simulink model "MHILSimRef"  (R2021b)
settings: Solver=VariableStepAuto  StartTime=0.0  StopTime=1e-3  RelTol=1e-3
values from neighbouring files (symbols this model uses):
  m = tddbl_model    [HILSimModel.m]
undefined symbols (not defined in the file or in its folder): s
libraries: simulink x3
settings Model: Creator=berndorfer  LastModifiedBy=berndorfer

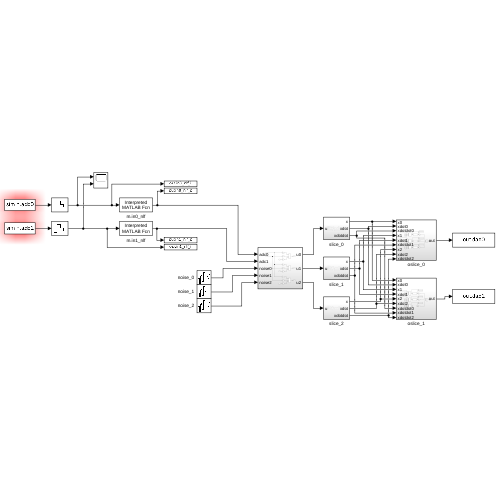
[thumbnail: Simulink's stored preview of the top-level diagram]
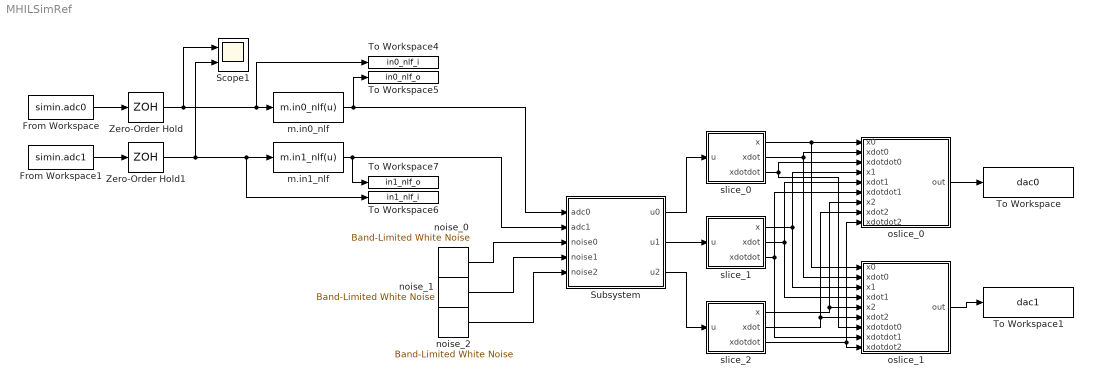
== system MHILSimRef ==
  From Workspace : FromWorkspace  VariableName=simin.adc0
  From Workspace1 : FromWorkspace  VariableName=simin.adc1
  Scope1 : Scope  NumInputPorts=2
  Subsystem : Subsystem
  To Workspace : ToWorkspace  VariableName=dac0  SaveFormat=Timeseries  SampleTime=-1
  To Workspace1 : ToWorkspace  VariableName=dac1  SaveFormat=Timeseries  SampleTime=-1
  To Workspace4 : ToWorkspace  VariableName=in0_nlf_i  SaveFormat=Timeseries  SampleTime=-1
  To Workspace5 : ToWorkspace  VariableName=in0_nlf_o  SaveFormat=Timeseries  SampleTime=-1
  To Workspace6 : ToWorkspace  VariableName=in1_nlf_i  SaveFormat=Timeseries  SampleTime=-1
  To Workspace7 : ToWorkspace  VariableName=in1_nlf_o  SaveFormat=Timeseries  SampleTime=-1
  Zero-Order Hold : ZeroOrderHold  SampleTime=m.t_s
  Zero-Order Hold1 : ZeroOrderHold  SampleTime=m.t_s
  m.in0_nlf : MATLABFcn  MATLABFcn=m.in0_nlf(u)  OutputDimensions=1
  m.in1_nlf : MATLABFcn  MATLABFcn=m.in1_nlf(u)  OutputDimensions=1
  noise_0 : simulink/Sources/Band-Limited White Noise  Cov=[m.n0_power*m.t_s]  Ts=m.t_s  seed=[23341]
  noise_1 : simulink/Sources/Band-Limited White Noise  Cov=[m.n1_power*m.t_s]  Ts=m.t_s  seed=[23341]
  noise_2 : simulink/Sources/Band-Limited White Noise  Cov=[m.n2_power*m.t_s]  Ts=m.t_s  seed=[23341]
  oslice_0 : Subsystem
  oslice_1 : Subsystem
  slice_0 : Subsystem
  slice_1 : Subsystem
  slice_2 : Subsystem
  wires:
  Subsystem/2(u1) -> slice_1/1(u)
  Subsystem/3(u2) -> slice_2/1(u)
  Subsystem/1(u0) -> slice_0/1(u)
  Zero-Order Hold/1 -> Scope1/1, To Workspace4/1, m.in0_nlf/1
  m.in1_nlf/1 -> Subsystem/2(adc1), To Workspace7/1
  noise_1/1 -> Subsystem/4(noise1)
  m.in0_nlf/1 -> Subsystem/1(adc0), To Workspace5/1
  noise_2/1 -> Subsystem/5(noise2)
  noise_0/1 -> Subsystem/3(noise0)
  Zero-Order Hold1/1 -> Scope1/2, To Workspace6/1, m.in1_nlf/1
  From Workspace/1 -> Zero-Order Hold/1
  From Workspace1/1 -> Zero-Order Hold1/1
  slice_1/1(x) -> oslice_1/3(x1), oslice_0/4(x1)
  slice_0/1(x) -> oslice_1/1(x0), oslice_0/1(x0)
  slice_2/2(xdot) -> oslice_0/8(xdot2), oslice_1/6(xdot2)
  slice_0/2(xdot) -> oslice_1/2(xdot0), oslice_0/2(xdot0)
  slice_2/1(x) -> oslice_1/5(x2), oslice_0/7(x2)
  slice_1/2(xdot) -> oslice_1/4(xdot1), oslice_0/5(xdot1)
  oslice_0/1(out) -> To Workspace/1
  oslice_1/1(out) -> To Workspace1/1
  slice_0/3(xdotdot) -> oslice_1/7(xdotdot0), oslice_0/3(xdotdot0)
  slice_1/3(xdotdot) -> oslice_1/8(xdotdot1), oslice_0/6(xdotdot1)
  slice_2/3(xdotdot) -> oslice_1/9(xdotdot2), oslice_0/9(xdotdot2)

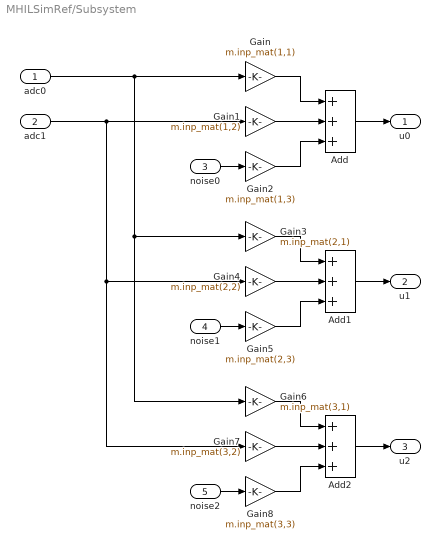
== system MHILSimRef/Subsystem ==
  adc0 : Inport
  adc1 : Inport  Port=2
  noise0 : Inport  Port=3
  noise1 : Inport  Port=4
  noise2 : Inport  Port=5
  Add : Sum  Inputs=+++
  Add1 : Sum  Inputs=+++
  Add2 : Sum  Inputs=+++
  Gain : Gain  Gain=m.inp_mat(1,1)
  Gain1 : Gain  Gain=m.inp_mat(1,2)
  Gain2 : Gain  Gain=m.inp_mat(1,3)
  Gain3 : Gain  Gain=m.inp_mat(2,1)
  Gain4 : Gain  Gain=m.inp_mat(2,2)
  Gain5 : Gain  Gain=m.inp_mat(2,3)
  Gain6 : Gain  Gain=m.inp_mat(3,1)
  Gain7 : Gain  Gain=m.inp_mat(3,2)
  Gain8 : Gain  Gain=m.inp_mat(3,3)
  u0 : Outport
  u1 : Outport  Port=2
  u2 : Outport  Port=3
  wires:
  adc0/1 -> Gain6/1, Gain3/1, Gain/1
  adc1/1 -> Gain7/1, Gain4/1, Gain1/1
  noise0/1 -> Gain2/1
  Gain1/1 -> Add/2
  Gain/1 -> Add/1
  Gain2/1 -> Add/3
  Add/1 -> u0/1
  noise1/1 -> Gain5/1
  Gain4/1 -> Add1/2
  Gain3/1 -> Add1/1
  Gain5/1 -> Add1/3
  Add1/1 -> u1/1
  noise2/1 -> Gain8/1
  Gain7/1 -> Add2/2
  Gain6/1 -> Add2/1
  Gain8/1 -> Add2/3
  Add2/1 -> u2/1

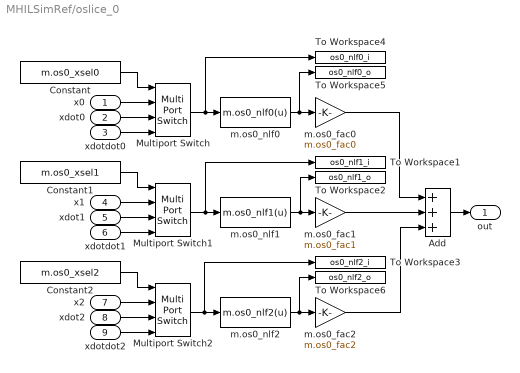
== system MHILSimRef/oslice_0 ==
  x0 : Inport
  xdot0 : Inport  Port=2
  xdotdot0 : Inport  Port=3
  x1 : Inport  Port=4
  xdot1 : Inport  Port=5
  xdotdot1 : Inport  Port=6
  x2 : Inport  Port=7
  xdot2 : Inport  Port=8
  xdotdot2 : Inport  Port=9
  Add : Sum  Inputs=+++
  Constant : Constant  Value=m.os0_xsel0
  Constant1 : Constant  Value=m.os0_xsel1
  Constant2 : Constant  Value=m.os0_xsel2
  Multiport Switch : MultiPortSwitch  DataPortOrder=Zero-based contiguous  zeroidx=on
  Multiport Switch1 : MultiPortSwitch  DataPortOrder=Zero-based contiguous  zeroidx=on
  Multiport Switch2 : MultiPortSwitch  DataPortOrder=Zero-based contiguous  zeroidx=on
  To Workspace1 : ToWorkspace  VariableName=os0_nlf1_i  SaveFormat=Timeseries  SampleTime=-1
  To Workspace2 : ToWorkspace  VariableName=os0_nlf1_o  SaveFormat=Timeseries  SampleTime=-1
  To Workspace3 : ToWorkspace  VariableName=os0_nlf2_i  SaveFormat=Timeseries  SampleTime=-1
  To Workspace4 : ToWorkspace  VariableName=os0_nlf0_i  SaveFormat=Timeseries  SampleTime=-1
  To Workspace5 : ToWorkspace  VariableName=os0_nlf0_o  SaveFormat=Timeseries  SampleTime=-1
  To Workspace6 : ToWorkspace  VariableName=os0_nlf2_o  SaveFormat=Timeseries  SampleTime=-1
  m.os0_fac0 : Gain  Gain=m.os0_fac0
  m.os0_fac1 : Gain  Gain=m.os0_fac1
  m.os0_fac2 : Gain  Gain=m.os0_fac2
  m.os0_nlf0 : MATLABFcn  MATLABFcn=m.os0_nlf0(u)  OutputDimensions=1
  m.os0_nlf1 : MATLABFcn  MATLABFcn=m.os0_nlf1(u)  OutputDimensions=1
  m.os0_nlf2 : MATLABFcn  MATLABFcn=m.os0_nlf2(u)  OutputDimensions=1
  out : Outport
  wires:
  m.os0_nlf0/1 -> To Workspace5/1, m.os0_fac0/1
  Multiport Switch1/1 -> To Workspace1/1, m.os0_nlf1/1
  Multiport Switch2/1 -> To Workspace3/1, m.os0_nlf2/1
  m.os0_nlf1/1 -> To Workspace2/1, m.os0_fac1/1
  m.os0_nlf2/1 -> To Workspace6/1, m.os0_fac2/1
  m.os0_fac1/1 -> Add/2
  Add/1 -> out/1
  m.os0_fac0/1 -> Add/1
  m.os0_fac2/1 -> Add/3
  xdot0/1 -> Multiport Switch/3
  x0/1 -> Multiport Switch/2
  Multiport Switch/1 -> To Workspace4/1, m.os0_nlf0/1
  Constant/1 -> Multiport Switch/1
  xdotdot0/1 -> Multiport Switch/4
  xdot1/1 -> Multiport Switch1/3
  x1/1 -> Multiport Switch1/2
  xdotdot1/1 -> Multiport Switch1/4
  Constant1/1 -> Multiport Switch1/1
  Constant2/1 -> Multiport Switch2/1
  xdot2/1 -> Multiport Switch2/3
  xdotdot2/1 -> Multiport Switch2/4
  x2/1 -> Multiport Switch2/2

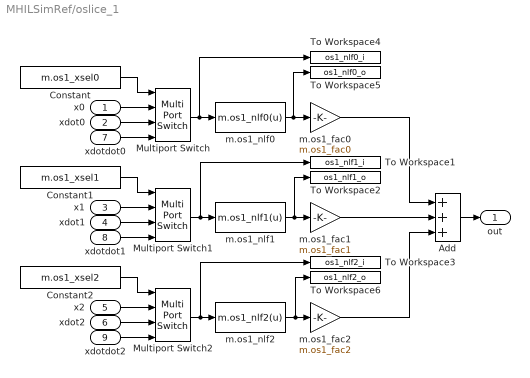
== system MHILSimRef/oslice_1 ==
  x0 : Inport
  xdot0 : Inport  Port=2
  x1 : Inport  Port=3
  xdot1 : Inport  Port=4
  x2 : Inport  Port=5
  xdot2 : Inport  Port=6
  xdotdot0 : Inport  Port=7
  xdotdot1 : Inport  Port=8
  xdotdot2 : Inport  Port=9
  Add : Sum  Inputs=+++
  Constant : Constant  Value=m.os1_xsel0
  Constant1 : Constant  Value=m.os1_xsel1
  Constant2 : Constant  Value=m.os1_xsel2
  Multiport Switch : MultiPortSwitch  DataPortOrder=Zero-based contiguous  zeroidx=on
  Multiport Switch1 : MultiPortSwitch  DataPortOrder=Zero-based contiguous  zeroidx=on
  Multiport Switch2 : MultiPortSwitch  DataPortOrder=Zero-based contiguous  zeroidx=on
  To Workspace1 : ToWorkspace  VariableName=os1_nlf1_i  SaveFormat=Timeseries  SampleTime=-1
  To Workspace2 : ToWorkspace  VariableName=os1_nlf1_o  SaveFormat=Timeseries  SampleTime=-1
  To Workspace3 : ToWorkspace  VariableName=os1_nlf2_i  SaveFormat=Timeseries  SampleTime=-1
  To Workspace4 : ToWorkspace  VariableName=os1_nlf0_i  SaveFormat=Timeseries  SampleTime=-1
  To Workspace5 : ToWorkspace  VariableName=os1_nlf0_o  SaveFormat=Timeseries  SampleTime=-1
  To Workspace6 : ToWorkspace  VariableName=os1_nlf2_o  SaveFormat=Timeseries  SampleTime=-1
  m.os1_fac0 : Gain  Gain=m.os1_fac0
  m.os1_fac1 : Gain  Gain=m.os1_fac1
  m.os1_fac2 : Gain  Gain=m.os1_fac2
  m.os1_nlf0 : MATLABFcn  MATLABFcn=m.os1_nlf0(u)  OutputDimensions=1
  m.os1_nlf1 : MATLABFcn  MATLABFcn=m.os1_nlf1(u)  OutputDimensions=1
  m.os1_nlf2 : MATLABFcn  MATLABFcn=m.os1_nlf2(u)  OutputDimensions=1
  out : Outport
  wires:
  Multiport Switch/1 -> To Workspace4/1, m.os1_nlf0/1
  m.os1_nlf0/1 -> To Workspace5/1, m.os1_fac0/1
  Multiport Switch1/1 -> To Workspace1/1, m.os1_nlf1/1
  Multiport Switch2/1 -> To Workspace3/1, m.os1_nlf2/1
  m.os1_nlf1/1 -> To Workspace2/1, m.os1_fac1/1
  m.os1_fac1/1 -> Add/2
  Add/1 -> out/1
  m.os1_fac0/1 -> Add/1
  m.os1_fac2/1 -> Add/3
  m.os1_nlf2/1 -> To Workspace6/1, m.os1_fac2/1
  x2/1 -> Multiport Switch2/2
  xdotdot2/1 -> Multiport Switch2/4
  xdot0/1 -> Multiport Switch/3
  x0/1 -> Multiport Switch/2
  xdot2/1 -> Multiport Switch2/3
  Constant1/1 -> Multiport Switch1/1
  Constant2/1 -> Multiport Switch2/1
  xdot1/1 -> Multiport Switch1/3
  xdotdot1/1 -> Multiport Switch1/4
  xdotdot0/1 -> Multiport Switch/4
  Constant/1 -> Multiport Switch/1
  x1/1 -> Multiport Switch1/2

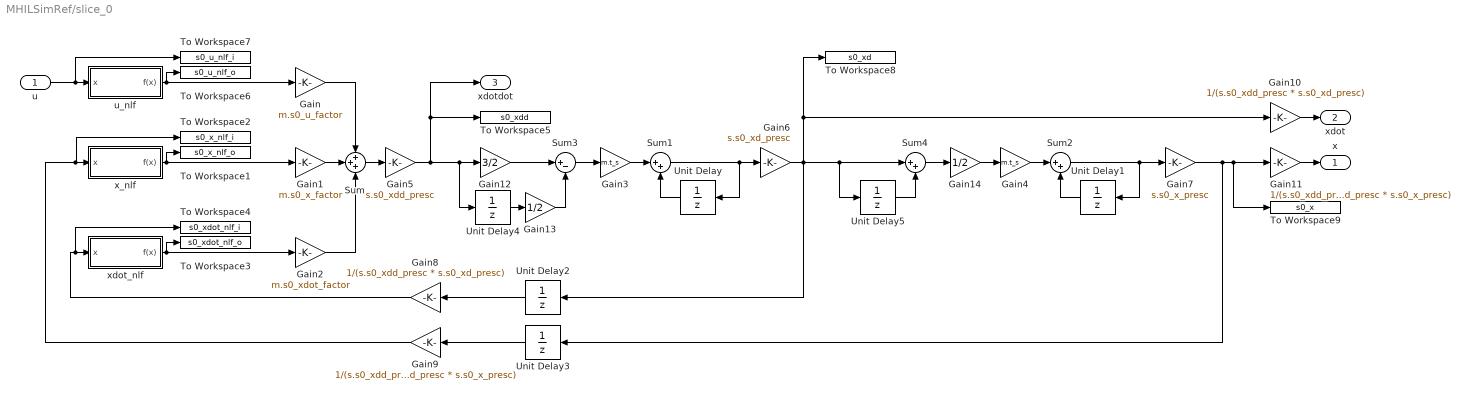
== system MHILSimRef/slice_0 ==
  u : Inport
  Gain : Gain  Gain=m.s0_u_factor
  Gain1 : Gain  Gain=m.s0_x_factor
  Gain10 : Gain  Gain=1/(s.s0_xdd_presc * s.s0_xd_presc)
  Gain11 : Gain  Gain=1/(s.s0_xdd_presc * s.s0_xd_presc * s.s0_x_presc)
  Gain12 : Gain  Gain=3/2
  Gain13 : Gain  Gain=1/2
  Gain14 : Gain  Gain=1/2
  Gain2 : Gain  Gain=m.s0_xdot_factor
  Gain3 : Gain  Gain=m.t_s
  Gain4 : Gain  Gain=m.t_s
  Gain5 : Gain  Gain=s.s0_xdd_presc
  Gain6 : Gain  Gain=s.s0_xd_presc
  Gain7 : Gain  Gain=s.s0_x_presc
  Gain8 : Gain  Gain=1/(s.s0_xdd_presc * s.s0_xd_presc)
  Gain9 : Gain  Gain=1/(s.s0_xdd_presc * s.s0_xd_presc * s.s0_x_presc)
  Sum : Sum  Inputs=+++
  Sum1 : Sum  Inputs=|++
  Sum2 : Sum  Inputs=|++
  Sum3 : Sum  Inputs=|+-
  Sum4 : Sum  Inputs=|++
  To Workspace1 : ToWorkspace  VariableName=s0_x_nlf_o  SaveFormat=Timeseries  SampleTime=-1
  To Workspace2 : ToWorkspace  VariableName=s0_x_nlf_i  SaveFormat=Timeseries  SampleTime=-1
  To Workspace3 : ToWorkspace  VariableName=s0_xdot_nlf_o  SaveFormat=Timeseries  SampleTime=-1
  To Workspace4 : ToWorkspace  VariableName=s0_xdot_nlf_i  SaveFormat=Timeseries  SampleTime=-1
  To Workspace5 : ToWorkspace  VariableName=s0_xdd  SaveFormat=Timeseries  SampleTime=-1
  To Workspace6 : ToWorkspace  VariableName=s0_u_nlf_o  SaveFormat=Timeseries  SampleTime=-1
  To Workspace7 : ToWorkspace  VariableName=s0_u_nlf_i  SaveFormat=Timeseries  SampleTime=-1
  To Workspace8 : ToWorkspace  VariableName=s0_xd  SaveFormat=Timeseries  SampleTime=-1
  To Workspace9 : ToWorkspace  VariableName=s0_x  SaveFormat=Timeseries  SampleTime=-1
  Unit Delay{,1..5} (6 alike) : UnitDelay  SampleTime=m.t_s  HasFrameUpgradeWarning=on
  u_nlf : Subsystem
  x_nlf : Subsystem
  xdot_nlf : Subsystem
  x : Outport
  xdot : Outport  Port=2
  xdotdot : Outport  Port=3
  wires:
  u/1 -> u_nlf/1(x), To Workspace7/1
  u_nlf/1(f(x)) -> Gain/1, To Workspace6/1
  Gain1/1 -> Sum/2
  Gain2/1 -> Sum/3
  Gain/1 -> Sum/1
  Unit Delay/1 -> Sum1/2
  Sum1/1 -> Gain6/1, Unit Delay/1
  Sum2/1 -> Gain7/1, Unit Delay1/1
  Unit Delay1/1 -> Sum2/2
  Gain3/1 -> Sum1/1
  Gain4/1 -> Sum2/1
  Unit Delay3/1 -> Gain9/1
  x_nlf/1(f(x)) -> To Workspace1/1, Gain1/1
  Unit Delay2/1 -> Gain8/1
  xdot_nlf/1(f(x)) -> To Workspace3/1, Gain2/1
  Sum/1 -> Gain5/1
  Gain7/1 -> Unit Delay3/1, Gain11/1, To Workspace9/1
  Gain8/1 -> xdot_nlf/1(x), To Workspace4/1
  Gain9/1 -> To Workspace2/1, x_nlf/1(x)
  Gain10/1 -> xdot/1
  Gain11/1 -> x/1
  Gain12/1 -> Sum3/1
  Gain5/1 -> Unit Delay4/1, Gain12/1, xdotdot/1, To Workspace5/1
  Unit Delay4/1 -> Gain13/1
  Sum3/1 -> Gain3/1
  Gain13/1 -> Sum3/2
  Gain6/1 -> Unit Delay5/1, Sum4/1, To Workspace8/1, Gain10/1, Unit Delay2/1
  Sum4/1 -> Gain14/1
  Unit Delay5/1 -> Sum4/2
  Gain14/1 -> Gain4/1

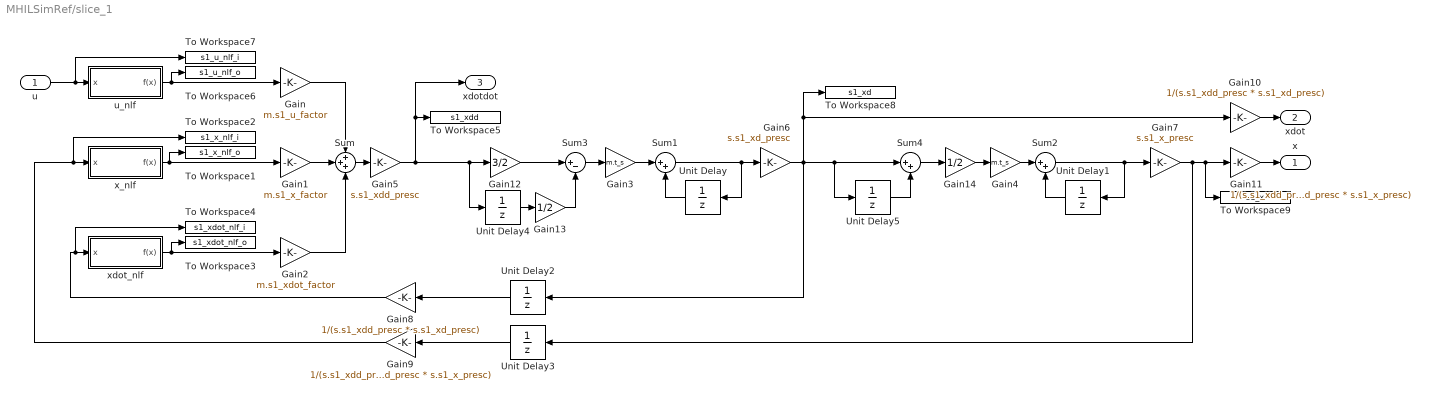
== system MHILSimRef/slice_1 ==
  u : Inport
  Gain : Gain  Gain=m.s1_u_factor
  Gain1 : Gain  Gain=m.s1_x_factor
  Gain10 : Gain  Gain=1/(s.s1_xdd_presc * s.s1_xd_presc)
  Gain11 : Gain  Gain=1/(s.s1_xdd_presc * s.s1_xd_presc * s.s1_x_presc)
  Gain12 : Gain  Gain=3/2
  Gain13 : Gain  Gain=1/2
  Gain14 : Gain  Gain=1/2
  Gain2 : Gain  Gain=m.s1_xdot_factor
  Gain3 : Gain  Gain=m.t_s
  Gain4 : Gain  Gain=m.t_s
  Gain5 : Gain  Gain=s.s1_xdd_presc
  Gain6 : Gain  Gain=s.s1_xd_presc
  Gain7 : Gain  Gain=s.s1_x_presc
  Gain8 : Gain  Gain=1/(s.s1_xdd_presc * s.s1_xd_presc)
  Gain9 : Gain  Gain=1/(s.s1_xdd_presc * s.s1_xd_presc * s.s1_x_presc)
  Sum : Sum  Inputs=+++
  Sum1 : Sum  Inputs=|++
  Sum2 : Sum  Inputs=|++
  Sum3 : Sum  Inputs=|+-
  Sum4 : Sum  Inputs=|++
  To Workspace1 : ToWorkspace  VariableName=s1_x_nlf_o  SaveFormat=Timeseries  SampleTime=-1
  To Workspace2 : ToWorkspace  VariableName=s1_x_nlf_i  SaveFormat=Timeseries  SampleTime=-1
  To Workspace3 : ToWorkspace  VariableName=s1_xdot_nlf_o  SaveFormat=Timeseries  SampleTime=-1
  To Workspace4 : ToWorkspace  VariableName=s1_xdot_nlf_i  SaveFormat=Timeseries  SampleTime=-1
  To Workspace5 : ToWorkspace  VariableName=s1_xdd  SaveFormat=Timeseries  SampleTime=-1
  To Workspace6 : ToWorkspace  VariableName=s1_u_nlf_o  SaveFormat=Timeseries  SampleTime=-1
  To Workspace7 : ToWorkspace  VariableName=s1_u_nlf_i  SaveFormat=Timeseries  SampleTime=-1
  To Workspace8 : ToWorkspace  VariableName=s1_xd  SaveFormat=Timeseries  SampleTime=-1
  To Workspace9 : ToWorkspace  VariableName=s1_x  SaveFormat=Timeseries  SampleTime=-1
  Unit Delay{,1..5} (6 alike) : UnitDelay  SampleTime=m.t_s  HasFrameUpgradeWarning=on
  u_nlf : Subsystem
  x_nlf : Subsystem
  xdot_nlf : Subsystem
  x : Outport
  xdot : Outport  Port=2
  xdotdot : Outport  Port=3
  wires:
  Gain1/1 -> Sum/2
  Gain2/1 -> Sum/3
  Gain/1 -> Sum/1
  Sum/1 -> Gain5/1
  Unit Delay/1 -> Sum1/2
  Sum1/1 -> Gain6/1, Unit Delay/1
  Sum2/1 -> Gain7/1, Unit Delay1/1
  Unit Delay1/1 -> Sum2/2
  Gain3/1 -> Sum1/1
  Gain4/1 -> Sum2/1
  u/1 -> u_nlf/1(x), To Workspace7/1
  u_nlf/1(f(x)) -> To Workspace6/1, Gain/1
  x_nlf/1(f(x)) -> To Workspace1/1, Gain1/1
  Unit Delay3/1 -> Gain9/1
  xdot_nlf/1(f(x)) -> To Workspace3/1, Gain2/1
  Unit Delay2/1 -> Gain8/1
  Gain7/1 -> Unit Delay3/1, Gain11/1, To Workspace9/1
  Gain8/1 -> xdot_nlf/1(x), To Workspace4/1
  Gain9/1 -> x_nlf/1(x), To Workspace2/1
  Gain10/1 -> xdot/1
  Gain11/1 -> x/1
  Gain12/1 -> Sum3/1
  Sum3/1 -> Gain3/1
  Gain13/1 -> Sum3/2
  Unit Delay4/1 -> Gain13/1
  Sum4/1 -> Gain14/1
  Gain6/1 -> Unit Delay5/1, Sum4/1, Gain10/1, To Workspace8/1, Unit Delay2/1
  Gain14/1 -> Gain4/1
  Unit Delay5/1 -> Sum4/2
  Gain5/1 -> Unit Delay4/1, Gain12/1, xdotdot/1, To Workspace5/1

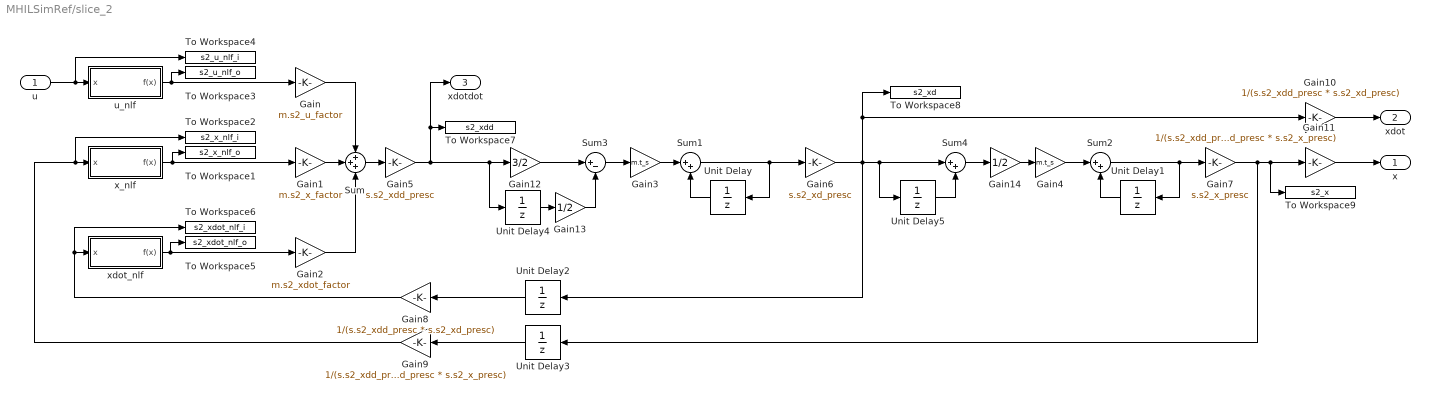
== system MHILSimRef/slice_2 ==
  u : Inport
  Gain : Gain  Gain=m.s2_u_factor
  Gain1 : Gain  Gain=m.s2_x_factor
  Gain10 : Gain  Gain=1/(s.s2_xdd_presc * s.s2_xd_presc)
  Gain11 : Gain  Gain=1/(s.s2_xdd_presc * s.s2_xd_presc * s.s2_x_presc)
  Gain12 : Gain  Gain=3/2
  Gain13 : Gain  Gain=1/2
  Gain14 : Gain  Gain=1/2
  Gain2 : Gain  Gain=m.s2_xdot_factor
  Gain3 : Gain  Gain=m.t_s
  Gain4 : Gain  Gain=m.t_s
  Gain5 : Gain  Gain=s.s2_xdd_presc
  Gain6 : Gain  Gain=s.s2_xd_presc
  Gain7 : Gain  Gain=s.s2_x_presc
  Gain8 : Gain  Gain=1/(s.s2_xdd_presc * s.s2_xd_presc)
  Gain9 : Gain  Gain=1/(s.s2_xdd_presc * s.s2_xd_presc * s.s2_x_presc)
  Sum : Sum  Inputs=+++
  Sum1 : Sum  Inputs=|++
  Sum2 : Sum  Inputs=|++
  Sum3 : Sum  Inputs=|+-
  Sum4 : Sum  Inputs=|++
  To Workspace1 : ToWorkspace  VariableName=s2_x_nlf_o  SaveFormat=Timeseries  SampleTime=-1
  To Workspace2 : ToWorkspace  VariableName=s2_x_nlf_i  SaveFormat=Timeseries  SampleTime=-1
  To Workspace3 : ToWorkspace  VariableName=s2_u_nlf_o  SaveFormat=Timeseries  SampleTime=-1
  To Workspace4 : ToWorkspace  VariableName=s2_u_nlf_i  SaveFormat=Timeseries  SampleTime=-1
  To Workspace5 : ToWorkspace  VariableName=s2_xdot_nlf_o  SaveFormat=Timeseries  SampleTime=-1
  To Workspace6 : ToWorkspace  VariableName=s2_xdot_nlf_i  SaveFormat=Timeseries  SampleTime=-1
  To Workspace7 : ToWorkspace  VariableName=s2_xdd  SaveFormat=Timeseries  SampleTime=-1
  To Workspace8 : ToWorkspace  VariableName=s2_xd  SaveFormat=Timeseries  SampleTime=-1
  To Workspace9 : ToWorkspace  VariableName=s2_x  SaveFormat=Timeseries  SampleTime=-1
  Unit Delay{,1..5} (6 alike) : UnitDelay  SampleTime=m.t_s  HasFrameUpgradeWarning=on
  u_nlf : Subsystem
  x_nlf : Subsystem
  xdot_nlf : Subsystem
  x : Outport
  xdot : Outport  Port=2
  xdotdot : Outport  Port=3
  wires:
  Gain1/1 -> Sum/2
  Gain2/1 -> Sum/3
  Gain/1 -> Sum/1
  Sum/1 -> Gain5/1
  Unit Delay/1 -> Sum1/2
  Sum1/1 -> Gain6/1, Unit Delay/1
  Sum2/1 -> Gain7/1, Unit Delay1/1
  Unit Delay1/1 -> Sum2/2
  Gain3/1 -> Sum1/1
  Gain4/1 -> Sum2/1
  u_nlf/1(f(x)) -> To Workspace3/1, Gain/1
  u/1 -> u_nlf/1(x), To Workspace4/1
  x_nlf/1(f(x)) -> To Workspace1/1, Gain1/1
  Unit Delay3/1 -> Gain9/1
  xdot_nlf/1(f(x)) -> To Workspace5/1, Gain2/1
  Unit Delay2/1 -> Gain8/1
  Gain7/1 -> Unit Delay3/1, Gain11/1, To Workspace9/1
  Gain8/1 -> xdot_nlf/1(x), To Workspace6/1
  Gain9/1 -> x_nlf/1(x), To Workspace2/1
  Gain10/1 -> xdot/1
  Gain11/1 -> x/1
  Gain12/1 -> Sum3/1
  Gain5/1 -> Unit Delay4/1, Gain12/1, xdotdot/1, To Workspace7/1
  Gain13/1 -> Sum3/2
  Unit Delay4/1 -> Gain13/1
  Sum3/1 -> Gain3/1
  Sum4/1 -> Gain14/1
  Gain6/1 -> Unit Delay5/1, Sum4/1, Gain10/1, To Workspace8/1, Unit Delay2/1
  Gain14/1 -> Gain4/1
  Unit Delay5/1 -> Sum4/2

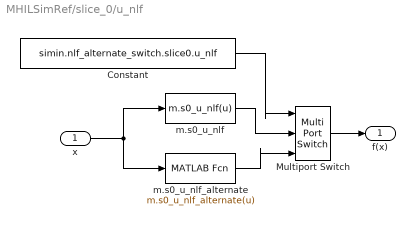
== system MHILSimRef/slice_0/u_nlf ==
  x : Inport
  Constant : Constant  Value=simin.nlf_alternate_switch.slice0.u_nlf
  Multiport Switch : MultiPortSwitch  DataPortOrder=Zero-based contiguous  Inputs=2  zeroidx=on
  m.s0_u_nlf : MATLABFcn  MATLABFcn=m.s0_u_nlf(u)  OutputDimensions=1
  m.s0_u_nlf_alternate : MATLABFcn  MATLABFcn=m.s0_u_nlf_alternate(u)  OutputDimensions=1
  f(x) : Outport
  wires:
  m.s0_u_nlf/1 -> Multiport Switch/2
  m.s0_u_nlf_alternate/1 -> Multiport Switch/3
  Multiport Switch/1 -> f(x)/1
  x/1 -> m.s0_u_nlf/1, m.s0_u_nlf_alternate/1
  Constant/1 -> Multiport Switch/1

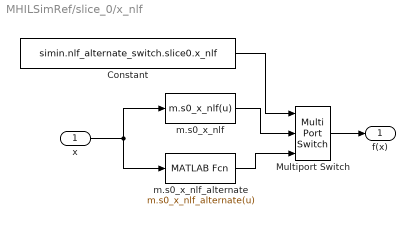
== system MHILSimRef/slice_0/x_nlf ==
  x : Inport
  Constant : Constant  Value=simin.nlf_alternate_switch.slice0.x_nlf
  Multiport Switch : MultiPortSwitch  DataPortOrder=Zero-based contiguous  Inputs=2  zeroidx=on
  m.s0_x_nlf : MATLABFcn  MATLABFcn=m.s0_x_nlf(u)  OutputDimensions=1
  m.s0_x_nlf_alternate : MATLABFcn  MATLABFcn=m.s0_x_nlf_alternate(u)  OutputDimensions=1
  f(x) : Outport
  wires:
  m.s0_x_nlf/1 -> Multiport Switch/2
  m.s0_x_nlf_alternate/1 -> Multiport Switch/3
  Multiport Switch/1 -> f(x)/1
  x/1 -> m.s0_x_nlf/1, m.s0_x_nlf_alternate/1
  Constant/1 -> Multiport Switch/1

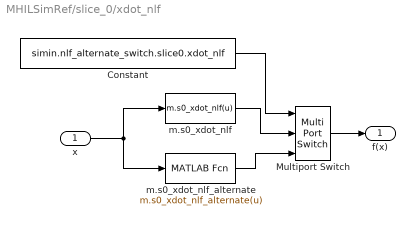
== system MHILSimRef/slice_0/xdot_nlf ==
  x : Inport
  Constant : Constant  Value=simin.nlf_alternate_switch.slice0.xdot_nlf
  Multiport Switch : MultiPortSwitch  DataPortOrder=Zero-based contiguous  Inputs=2  zeroidx=on
  m.s0_xdot_nlf : MATLABFcn  MATLABFcn=m.s0_xdot_nlf(u)  OutputDimensions=1
  m.s0_xdot_nlf_alternate : MATLABFcn  MATLABFcn=m.s0_xdot_nlf_alternate(u)  OutputDimensions=1
  f(x) : Outport
  wires:
  m.s0_xdot_nlf/1 -> Multiport Switch/2
  m.s0_xdot_nlf_alternate/1 -> Multiport Switch/3
  Multiport Switch/1 -> f(x)/1
  x/1 -> m.s0_xdot_nlf/1, m.s0_xdot_nlf_alternate/1
  Constant/1 -> Multiport Switch/1

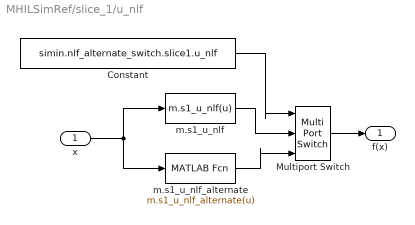
== system MHILSimRef/slice_1/u_nlf ==
  x : Inport
  Constant : Constant  Value=simin.nlf_alternate_switch.slice1.u_nlf
  Multiport Switch : MultiPortSwitch  DataPortOrder=Zero-based contiguous  Inputs=2  zeroidx=on
  m.s1_u_nlf : MATLABFcn  MATLABFcn=m.s1_u_nlf(u)  OutputDimensions=1
  m.s1_u_nlf_alternate : MATLABFcn  MATLABFcn=m.s1_u_nlf_alternate(u)  OutputDimensions=1
  f(x) : Outport
  wires:
  m.s1_u_nlf/1 -> Multiport Switch/2
  m.s1_u_nlf_alternate/1 -> Multiport Switch/3
  Multiport Switch/1 -> f(x)/1
  x/1 -> m.s1_u_nlf/1, m.s1_u_nlf_alternate/1
  Constant/1 -> Multiport Switch/1

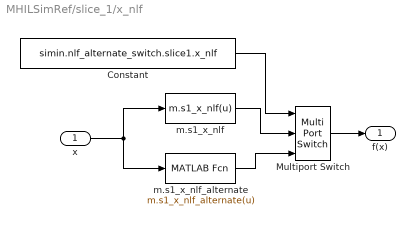
== system MHILSimRef/slice_1/x_nlf ==
  x : Inport
  Constant : Constant  Value=simin.nlf_alternate_switch.slice1.x_nlf
  Multiport Switch : MultiPortSwitch  DataPortOrder=Zero-based contiguous  Inputs=2  zeroidx=on
  m.s1_x_nlf : MATLABFcn  MATLABFcn=m.s1_x_nlf(u)  OutputDimensions=1
  m.s1_x_nlf_alternate : MATLABFcn  MATLABFcn=m.s1_x_nlf_alternate(u)  OutputDimensions=1
  f(x) : Outport
  wires:
  m.s1_x_nlf/1 -> Multiport Switch/2
  m.s1_x_nlf_alternate/1 -> Multiport Switch/3
  Multiport Switch/1 -> f(x)/1
  x/1 -> m.s1_x_nlf/1, m.s1_x_nlf_alternate/1
  Constant/1 -> Multiport Switch/1

== system MHILSimRef/slice_1/xdot_nlf ==
  x : Inport
  Constant : Constant  Value=simin.nlf_alternate_switch.slice1.xdot_nlf
  Multiport Switch : MultiPortSwitch  DataPortOrder=Zero-based contiguous  Inputs=2  zeroidx=on
  m.s1_xdot_nlf : MATLABFcn  MATLABFcn=m.s1_xdot_nlf(u)  OutputDimensions=1
  m.s1_xdot_nlf_alternate : MATLABFcn  MATLABFcn=m.s1_xdot_nlf_alternate(u)  OutputDimensions=1
  f(x) : Outport
  wires:
  m.s1_xdot_nlf/1 -> Multiport Switch/2
  m.s1_xdot_nlf_alternate/1 -> Multiport Switch/3
  Multiport Switch/1 -> f(x)/1
  x/1 -> m.s1_xdot_nlf/1, m.s1_xdot_nlf_alternate/1
  Constant/1 -> Multiport Switch/1

== system MHILSimRef/slice_2/u_nlf ==
  x : Inport
  Constant : Constant  Value=simin.nlf_alternate_switch.slice2.u_nlf
  Multiport Switch : MultiPortSwitch  DataPortOrder=Zero-based contiguous  Inputs=2  zeroidx=on
  m.s2_u_nlf : MATLABFcn  MATLABFcn=m.s2_u_nlf(u)  OutputDimensions=1
  m.s2_u_nlf_alternate : MATLABFcn  MATLABFcn=m.s2_u_nlf_alternate(u)  OutputDimensions=1
  f(x) : Outport
  wires:
  m.s2_u_nlf/1 -> Multiport Switch/2
  m.s2_u_nlf_alternate/1 -> Multiport Switch/3
  Multiport Switch/1 -> f(x)/1
  x/1 -> m.s2_u_nlf/1, m.s2_u_nlf_alternate/1
  Constant/1 -> Multiport Switch/1

== system MHILSimRef/slice_2/x_nlf ==
  x : Inport
  Constant : Constant  Value=simin.nlf_alternate_switch.slice2.x_nlf
  Multiport Switch : MultiPortSwitch  DataPortOrder=Zero-based contiguous  Inputs=2  zeroidx=on
  m.s2_x_nlf : MATLABFcn  MATLABFcn=m.s2_x_nlf(u)  OutputDimensions=1
  m.s2_x_nlf_alternate : MATLABFcn  MATLABFcn=m.s2_x_nlf_alternate(u)  OutputDimensions=1
  f(x) : Outport
  wires:
  m.s2_x_nlf/1 -> Multiport Switch/2
  m.s2_x_nlf_alternate/1 -> Multiport Switch/3
  Multiport Switch/1 -> f(x)/1
  x/1 -> m.s2_x_nlf/1, m.s2_x_nlf_alternate/1
  Constant/1 -> Multiport Switch/1

== system MHILSimRef/slice_2/xdot_nlf ==
  x : Inport
  Constant : Constant  Value=simin.nlf_alternate_switch.slice2.xdot_nlf
  Multiport Switch : MultiPortSwitch  DataPortOrder=Zero-based contiguous  Inputs=2  zeroidx=on
  m.s2_xdot_nlf : MATLABFcn  MATLABFcn=m.s2_xdot_nlf(u)  OutputDimensions=1
  m.s2_xdot_nlf_alternate : MATLABFcn  MATLABFcn=m.s2_xdot_nlf_alternate(u)  OutputDimensions=1
  f(x) : Outport
  wires:
  m.s2_xdot_nlf/1 -> Multiport Switch/2
  m.s2_xdot_nlf_alternate/1 -> Multiport Switch/3
  Multiport Switch/1 -> f(x)/1
  x/1 -> m.s2_xdot_nlf/1, m.s2_xdot_nlf_alternate/1
  Constant/1 -> Multiport Switch/1
